simulink model "Main_Sim_testingDesat"  (R2018b)
settings: Solver=FixedStepAuto  StartTime=0.0  StopTime=18000  FixedStep=simParams.sample_time_s  RelTol=1e-3  EnableMultiTasking=on
libraries: actuators_lib x1, CDH_command_lib x1, Environment_lib x1, FSW_Lib x1, Sensors_Lib x1, satelliteDynamics_lib x1
settings Model: Creator=devantormey  LastModifiedBy=colem
settings OptimizationCC: LifeSpan=inf
settings DebuggingCC: SFUnexpectedBacktrackingDiag=warning  SFNoUnconditionalDefaultTransitionDiag=warning
settings SFSimCC: SimUseLocalCustomCode=off
settings RTWCC: RTWUseLocalCustomCode=off
settings CodeAppCC: StateflowObjectComments=on
settings GRTTargetCC: TargetLangStandard=C89/C90 (ANSI)  GeneratePreprocessorConditionals=Disable all
settings ConfigComp: CovMetricSettings=dw  CovHtmlReporting=on  CovSaveCumulativeToWorkspaceVar=on  CovSaveSingleToWorkspaceVar=on  CovExternalEMLEnable=off

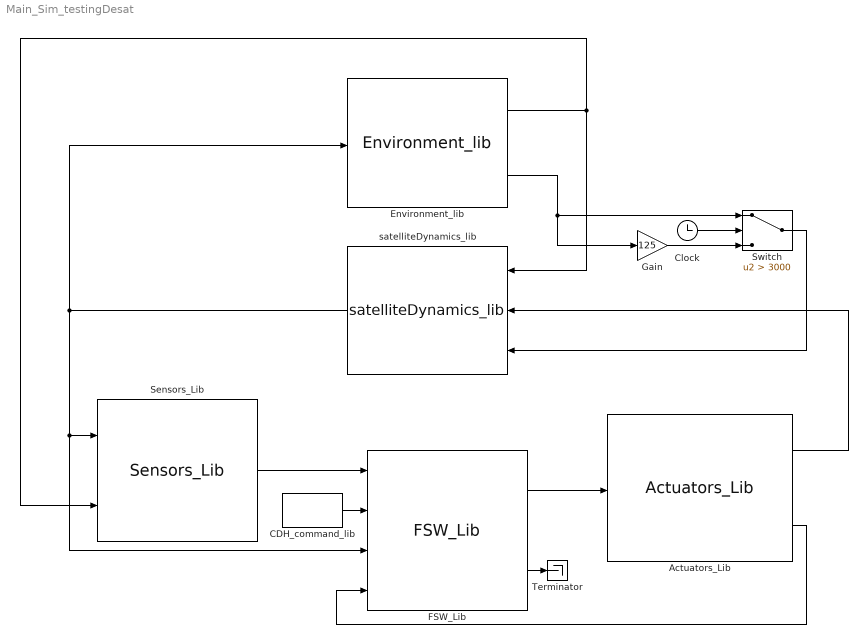
== system Main_Sim_testingDesat ==
  Actuators_Lib : actuators_lib/Actuators_Lib  SystemSampleTime=-1
  CDH_command_lib : CDH_command_lib/CDH_command_lib  SystemSampleTime=-1
  Clock : Clock
  Environment_lib : Environment_lib/Environment_lib  SystemSampleTime=-1
  FSW_Lib : FSW_Lib/FSW_Lib  SystemSampleTime=-1
  Gain : Gain  Gain=125
  Sensors_Lib : Sensors_Lib/Sensors_Lib  SystemSampleTime=-1
      link override Goto3: GotoTag=B_eci_T
  Switch : Switch  Criteria=u2 > Threshold  Threshold=3000
  Terminator : Terminator
  satelliteDynamics_lib : satelliteDynamics_lib/satelliteDynamics_lib  SystemSampleTime=-1
      link override "RigidBodyDynamics/Discrete-Time Integrator ": InitialCondition=simParams.initialConditions.w0.*[6;4;-3]*-2
  wires:
  FSW_Lib/1 -> Actuators_Lib/1
  Sensors_Lib/1 -> FSW_Lib/1
  satelliteDynamics_lib/1 -> Environment_lib/1, FSW_Lib/3, Sensors_Lib/1
  Environment_lib/1 -> Sensors_Lib/2, satelliteDynamics_lib/1
  Actuators_Lib/1 -> satelliteDynamics_lib/2
  FSW_Lib/2 -> Terminator/1
  Actuators_Lib/2 -> FSW_Lib/4
  CDH_command_lib/1 -> FSW_Lib/2
  Environment_lib/2 -> Switch/1, Gain/1
  Clock/1 -> Switch/2
  Gain/1 -> Switch/3
  Switch/1 -> satelliteDynamics_lib/3
